simulink model "PT3_mod"  (R2014a)
settings: Solver=ode45  StartTime=0.0  StopTime=10.0  RelTol=1e-3
values from neighbouring files (symbols this model uses):
  a1 = R * C1    (= 0.05307)    [PT3_dat.m]
  a2 = L*(C1 + C2)    (= 0.000412)    [PT3_dat.m]
  a3 = R*L*C1*C2    (= 1.263066e-05)    [PT3_dat.m]
  tstep = 1e-3    (= 0.001)    [PT3_dat.m]
  Uemax = 10    [PT3_dat.m]    (also in Uebung8.m = 2)
settings Model: Creator=wirth  LastModifiedBy=Uli
settings DataIOCC: SignalLoggingSaveFormat=ModelDataLogs
settings OptimizationCC: ExpressionDepthLimit=2147483647  InitFltsAndDblsToZero=on
settings DebuggingCC: UnderspecifiedInitializationDetection=Classic  FcnCallInpInsideContextMsg=UseLocalSettings  StateNameClashWarn=warning  StrictBusMsg=Warning
settings GRTTargetCC: CombineOutputUpdateFcns=off  GRTInterface=on

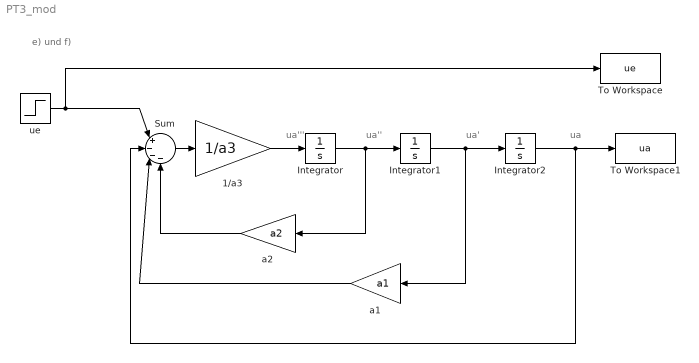
== system PT3_mod ==
  note: ua'''
  note: ua
  note: ua''
  note: ua'
  note: e) und f)
  1/a3 : Gain  Gain=1/a3
  Integrator : Integrator
  Integrator1 : Integrator
  Integrator2 : Integrator
  Sum : Sum  Inputs=|+---
  To Workspace : ToWorkspace  VariableName=ue  SampleTime=-1
  To Workspace1 : ToWorkspace  VariableName=ua  SampleTime=-1
  a1 : Gain  Gain=a1
  a2 : Gain  Gain=a2
  ue : Step  Time=tstep  After=Uemax  SampleTime=0
  wires:
  ue/1 -> To Workspace/1, Sum/1
  Integrator2/1 -> To Workspace1/1, Sum/2
  Integrator/1 -> Integrator1/1, a2/1
  Integrator1/1 -> Integrator2/1, a1/1
  a1/1 -> Sum/3
  a2/1 -> Sum/4
  1/a3/1 -> Integrator/1
  Sum/1 -> 1/a3/1
